simulink model "a1q3"  (R2021b)
settings: Solver=ode23t  StartTime=-0.1  StopTime=0.2  RelTol=1e-3
undefined symbols (not defined in the file or in its folder): denSim, numSim
settings Model: Creator=leos  LastModifiedBy=andre

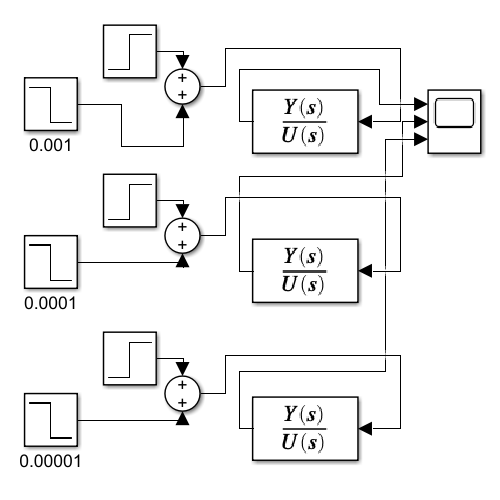
[thumbnail: Simulink's stored preview of the top-level diagram]
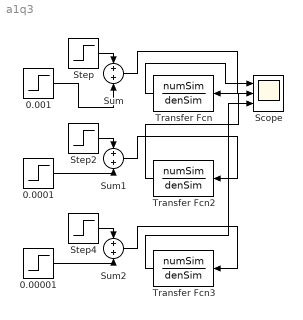
== system a1q3 ==
  0.00001 : Step  Time=0.00001  After=-100000  SampleTime=0
  0.0001 : Step  Time=0.0001  After=-10000  SampleTime=0
  0.001 : Step  Time=0.001  After=-1000  SampleTime=0
  Scope : Scope  NumInputPorts=3
  Step : Step  Time=0  After=1000  SampleTime=0
  Step2 : Step  Time=0  After=10000  SampleTime=0
  Step4 : Step  Time=0  After=100000  SampleTime=0
  Sum : Sum
  Sum1 : Sum
  Sum2 : Sum
  Transfer Fcn : TransferFcn  Numerator=numSim  Denominator=denSim
  Transfer Fcn2 : TransferFcn  Numerator=numSim  Denominator=denSim
  Transfer Fcn3 : TransferFcn  Numerator=numSim  Denominator=denSim
  wires:
  Step/1 -> Sum/1
  0.001/1 -> Sum/2
  Transfer Fcn/1 -> Scope/1
  Sum/1 -> Transfer Fcn/1
  Sum1/1 -> Transfer Fcn2/1
  Transfer Fcn2/1 -> Scope/2
  0.0001/1 -> Sum1/2
  Step2/1 -> Sum1/1
  Sum2/1 -> Transfer Fcn3/1
  Transfer Fcn3/1 -> Scope/3
  0.00001/1 -> Sum2/2
  Step4/1 -> Sum2/1
